simulink model "RM3ControlSim"  (R2015b)
settings: Solver=ode4  StartTime=0  StopTime=400  FixedStep=0.1  MaxStep=0.1  RelTol=1e-3
values from neighbouring files (symbols this model uses):
  simu = simulationClass()    [wecSimInputFile.m]
  waves = waveClass('irregular')    [wecSimInputFile.m]
undefined symbols (not defined in the file or in its folder): body, constraint, plant, pto, X, Y, Z
libraries: nesl_utility x72, vrlib x24, sm_lib x24, WECSim_Lib x3, simulink x2
(part 5 of 6)

== system RM3ControlSim/Rigid Body/Hydrodynamic Body/Morrison Element and ViscousDampingForceCalculation/Morrison Element Variant Subsystem/Morrison Element On/Regular Wave Morison Force/MorrisonElements/OrbitalVelocity ==
  Disp : Inport
  Time : Inport  Port=2
  MATLAB Function : MATLAB Function  TreatAsAtomicUnit=on
  WaveAmp : Constant  Value=waves.A(1,:)
  WaveFreq : Constant  Value=waves.w(1,:)
  WaveNumber : Constant  Value=waves.k(1,:)
  gravity : Constant  Value=simu.g  VectorParams1D=off
  phase : Constant  Value=0
  rampTime : Constant  Value=simu.rampTime  VectorParams1D=off
  waterDepth : Constant  Value=waves.waterDepth  VectorParams1D=off
  waveDirection : Constant  Value=waves.waveDir  VectorParams1D=off
  u-V : Outport
  w-V : Outport  Port=2
  u-A : Outport  Port=3
  w-A : Outport  Port=4
  v-V : Outport  Port=5
  v-A : Outport  Port=6
  wires:
  MATLAB Function/5(ya) -> v-A/1
  MATLAB Function/1(u) -> u-V/1
  MATLAB Function/2(v) -> v-V/1
  MATLAB Function/6(za) -> w-A/1
  MATLAB Function/4(xa) -> u-A/1
  MATLAB Function/3(w) -> w-V/1
  rampTime/1 -> MATLAB Function/7(rampT)
  waveDirection/1 -> MATLAB Function/8(waveDir)
  waterDepth/1 -> MATLAB Function/9(waterDepth)
  gravity/1 -> MATLAB Function/10(g)
  Time/1 -> MATLAB Function/6(time)
  WaveAmp/1 -> MATLAB Function/4(waveAmp)
  WaveFreq/1 -> MATLAB Function/3(waveFreq)
  WaveNumber/1 -> MATLAB Function/2(waveNumber)
  phase/1 -> MATLAB Function/5(randPhase)
  Disp/1 -> MATLAB Function/1(disp)

== system RM3ControlSim/Rigid Body/Hydrodynamic Body/Morrison Element and ViscousDampingForceCalculation/Morrison Element Variant Subsystem/Morrison Element On/Regular Wave Morison Force/MorrisonElements/Rotation1 ==
  rot1 : Inport
  rot2 : Inport  Port=2
  rot3 : Inport  Port=3
  2 : Product
  3 : Product  Inputs=3
  7 : Product
  8 : Product  Inputs=3
  Combine : Concatenate  NumInputs=3  Mode=Multidimensional array  ConcatenateDimension=2
  Trigonometric Function{,1..2,6,9,11} (6 alike) : Trigonometry  Operator=cos
  Trigonometric Function{3..5,7..8,10} (6 alike) : Trigonometry
  rot11 : Product
  rot12 : Sum
  rot13 : Sum  Inputs=+-
  rot[1,1-3] : Outport
  wires:
  rot13/1 -> Combine/3
  8/1 -> rot13/2
  7/1 -> rot13/1
  Trigonometric Function11/1 -> 8/3
  Trigonometric Function10/1 -> 8/2
  Trigonometric Function9/1 -> 8/1
  Trigonometric Function8/1 -> 7/2
  Trigonometric Function7/1 -> 7/1
  rot1/1 -> Trigonometric Function7/1, Trigonometric Function9/1, Trigonometric Function4/1, Trigonometric Function2/1
  rot3/1 -> Trigonometric Function8/1, Trigonometric Function11/1, Trigonometric Function6/1, Trigonometric Function3/1, Trigonometric Function1/1
  rot2/1 -> Trigonometric Function10/1, Trigonometric Function5/1, Trigonometric Function/1
  Combine/1 -> rot[1,1-3]/1
  rot12/1 -> Combine/2
  3/1 -> rot12/2
  2/1 -> rot12/1
  Trigonometric Function6/1 -> 3/3
  Trigonometric Function5/1 -> 3/2
  Trigonometric Function4/1 -> 3/1
  Trigonometric Function3/1 -> 2/2
  Trigonometric Function2/1 -> 2/1
  rot11/1 -> Combine/1
  Trigonometric Function1/1 -> rot11/2
  Trigonometric Function/1 -> rot11/1

== system RM3ControlSim/Rigid Body/Hydrodynamic Body/Morrison Element and ViscousDampingForceCalculation/Morrison Element Variant Subsystem/Morrison Element On/Regular Wave Morison Force/MorrisonElements/Rotation2 ==
  rot1 : Inport
  rot2 : Inport  Port=2
  rot3 : Inport  Port=3
  2 : Product
  3 : Product  Inputs=3
  7 : Product
  8 : Product  Inputs=3
  Combine : Concatenate  NumInputs=3  Mode=Multidimensional array  ConcatenateDimension=2
  Gain : Gain  Gain=-1
  Trigonometric Function{,2..3,8..9} (5 alike) : Trigonometry  Operator=cos
  Trigonometric Function{1,4..7,10..11} (7 alike) : Trigonometry
  rot11 : Product
  rot12 : Sum  Inputs=+-
  rot13 : Sum
  rot[2,1-3] : Outport
  wires:
  Gain/1 -> rot11/1
  rot13/1 -> Combine/3
  8/1 -> rot13/2
  7/1 -> rot13/1
  Trigonometric Function11/1 -> 8/3
  Trigonometric Function10/1 -> 8/2
  Trigonometric Function9/1 -> 8/1
  Trigonometric Function8/1 -> 7/2
  Trigonometric Function7/1 -> 7/1
  rot1/1 -> Trigonometric Function7/1, Trigonometric Function9/1, Trigonometric Function4/1, Trigonometric Function2/1
  rot3/1 -> Trigonometric Function8/1, Trigonometric Function11/1, Trigonometric Function6/1, Trigonometric Function3/1, Trigonometric Function1/1
  rot2/1 -> Trigonometric Function10/1, Trigonometric Function5/1, Trigonometric Function/1
  Combine/1 -> rot[2,1-3]/1
  rot12/1 -> Combine/2
  3/1 -> rot12/2
  2/1 -> rot12/1
  Trigonometric Function6/1 -> 3/3
  Trigonometric Function5/1 -> 3/2
  Trigonometric Function4/1 -> 3/1
  Trigonometric Function3/1 -> 2/2
  Trigonometric Function2/1 -> 2/1
  rot11/1 -> Combine/1
  Trigonometric Function1/1 -> rot11/2
  Trigonometric Function/1 -> Gain/1

== system RM3ControlSim/Rigid Body/Hydrodynamic Body/Morrison Element and ViscousDampingForceCalculation/Morrison Element Variant Subsystem/Morrison Element On/Regular Wave Morison Force/MorrisonElements/Rotation3 ==
  rot1 : Inport
  rot2 : Inport  Port=2
  2 : Product
  7 : Product
  Combine : Concatenate  NumInputs=3  Mode=Multidimensional array  ConcatenateDimension=2
  Gain1 : Gain  Gain=-1
  TrigFun1 : Trigonometry
  TrigFun2 : Trigonometry
  TrigFun3 : Trigonometry  Operator=cos
  TrigFun4 : Trigonometry  Operator=cos
  TrigFun5 : Trigonometry  Operator=cos
  rot[3,1-3] : Outport
  wires:
  Gain1/1 -> 2/1
  TrigFun2/1 -> Gain1/1
  7/1 -> Combine/3
  rot1/1 -> TrigFun4/1, TrigFun2/1
  TrigFun5/1 -> 7/2
  TrigFun4/1 -> 7/1
  rot2/1 -> TrigFun1/1, TrigFun3/1, TrigFun5/1
  Combine/1 -> rot[3,1-3]/1
  2/1 -> Combine/2
  TrigFun3/1 -> 2/2
  TrigFun1/1 -> Combine/1

== system RM3ControlSim/Rigid Body1/Hydrodynamic Body/Morrison Element and ViscousDampingForceCalculation/Morrison Element Variant Subsystem/Morrison Element On/Irregular Wave Morison Force/MorrisonElements/MorisonElementIrregular ==
  Disp : Inport
  waves.kirr : Inport  Port=2  Partition=on  PartitionDimension=1  PartitionWidth=1
  waves.w : Inport  Port=3  Partition=on  PartitionDimension=1  PartitionWidth=1
  waves.A : Inport  Port=4  Partition=on  PartitionDimension=1  PartitionWidth=1
  waves.RandPhase : Inport  Port=5  Partition=on  PartitionDimension=1  PartitionWidth=1
  Time : Inport  Port=6
  For Each : ForEach  DisableCoverage=on  IndexMode=One-based
  MATLAB Function : MATLAB Function  TreatAsAtomicUnit=on
  gravity : Constant  Value=simu.g  VectorParams1D=off
  rampTime : Constant  Value=simu.rampTime  VectorParams1D=off
  waterDepth : Constant  Value=waves.waterDepth  VectorParams1D=off
  waveDirection : Constant  Value=waves.waveDir  VectorParams1D=off
  u-V : Outport  ConcatenationDimension=1
  w-V : Outport  Port=2  ConcatenationDimension=1
  x-A : Outport  Port=3  ConcatenationDimension=1
  w-A : Outport  Port=4  ConcatenationDimension=1
  v-V : Outport  Port=5  ConcatenationDimension=1
  y-A : Outport  Port=6  ConcatenationDimension=1
  wires:
  MATLAB Function/3(w) -> w-V/1
  MATLAB Function/4(xa) -> x-A/1
  MATLAB Function/6(za) -> w-A/1
  MATLAB Function/5(ya) -> y-A/1
  MATLAB Function/2(v) -> v-V/1
  Time/1 -> MATLAB Function/6(time)
  waves.kirr/1 -> MATLAB Function/2(waveNumber)
  MATLAB Function/1(u) -> u-V/1
  waves.RandPhase/1 -> MATLAB Function/5(randPhase)
  waves.A/1 -> MATLAB Function/4(waveAmp)
  waves.w/1 -> MATLAB Function/3(waveFreq)
  Disp/1 -> MATLAB Function/1(disp)
  rampTime/1 -> MATLAB Function/7(rampT)
  waveDirection/1 -> MATLAB Function/8(waveDir)
  waterDepth/1 -> MATLAB Function/9(waterDepth)
  gravity/1 -> MATLAB Function/10(g)

== system RM3ControlSim/Rigid Body1/Hydrodynamic Body/Morrison Element and ViscousDampingForceCalculation/Morrison Element Variant Subsystem/Morrison Element On/Irregular Wave Morison Force/MorrisonElements/Rotation1 ==
  rot1 : Inport
  rot2 : Inport  Port=2
  rot3 : Inport  Port=3
  2 : Product
  3 : Product  Inputs=3
  7 : Product
  8 : Product  Inputs=3
  Combine : Concatenate  NumInputs=3  Mode=Multidimensional array  ConcatenateDimension=2
  Trigonometric Function{,1..2,6,9,11} (6 alike) : Trigonometry  Operator=cos
  Trigonometric Function{3..5,7..8,10} (6 alike) : Trigonometry
  rot11 : Product
  rot12 : Sum
  rot13 : Sum  Inputs=+-
  rot[1,1-3] : Outport
  wires:
  rot13/1 -> Combine/3
  8/1 -> rot13/2
  7/1 -> rot13/1
  Trigonometric Function11/1 -> 8/3
  Trigonometric Function10/1 -> 8/2
  Trigonometric Function9/1 -> 8/1
  Trigonometric Function8/1 -> 7/2
  Trigonometric Function7/1 -> 7/1
  rot1/1 -> Trigonometric Function7/1, Trigonometric Function9/1, Trigonometric Function4/1, Trigonometric Function2/1
  rot3/1 -> Trigonometric Function8/1, Trigonometric Function11/1, Trigonometric Function6/1, Trigonometric Function3/1, Trigonometric Function1/1
  rot2/1 -> Trigonometric Function10/1, Trigonometric Function5/1, Trigonometric Function/1
  Combine/1 -> rot[1,1-3]/1
  rot12/1 -> Combine/2
  3/1 -> rot12/2
  2/1 -> rot12/1
  Trigonometric Function6/1 -> 3/3
  Trigonometric Function5/1 -> 3/2
  Trigonometric Function4/1 -> 3/1
  Trigonometric Function3/1 -> 2/2
  Trigonometric Function2/1 -> 2/1
  rot11/1 -> Combine/1
  Trigonometric Function1/1 -> rot11/2
  Trigonometric Function/1 -> rot11/1

== system RM3ControlSim/Rigid Body1/Hydrodynamic Body/Morrison Element and ViscousDampingForceCalculation/Morrison Element Variant Subsystem/Morrison Element On/Irregular Wave Morison Force/MorrisonElements/Rotation2 ==
  rot1 : Inport
  rot2 : Inport  Port=2
  rot3 : Inport  Port=3
  2 : Product
  3 : Product  Inputs=3
  7 : Product
  8 : Product  Inputs=3
  Combine : Concatenate  NumInputs=3  Mode=Multidimensional array  ConcatenateDimension=2
  Gain : Gain  Gain=-1
  Trigonometric Function{,2..3,8..9} (5 alike) : Trigonometry  Operator=cos
  Trigonometric Function{1,4..7,10..11} (7 alike) : Trigonometry
  rot11 : Product
  rot12 : Sum  Inputs=+-
  rot13 : Sum
  rot[2,1-3] : Outport
  wires:
  Gain/1 -> rot11/1
  rot13/1 -> Combine/3
  8/1 -> rot13/2
  7/1 -> rot13/1
  Trigonometric Function11/1 -> 8/3
  Trigonometric Function10/1 -> 8/2
  Trigonometric Function9/1 -> 8/1
  Trigonometric Function8/1 -> 7/2
  Trigonometric Function7/1 -> 7/1
  rot1/1 -> Trigonometric Function7/1, Trigonometric Function9/1, Trigonometric Function4/1, Trigonometric Function2/1
  rot3/1 -> Trigonometric Function8/1, Trigonometric Function11/1, Trigonometric Function6/1, Trigonometric Function3/1, Trigonometric Function1/1
  rot2/1 -> Trigonometric Function10/1, Trigonometric Function5/1, Trigonometric Function/1
  Combine/1 -> rot[2,1-3]/1
  rot12/1 -> Combine/2
  3/1 -> rot12/2
  2/1 -> rot12/1
  Trigonometric Function6/1 -> 3/3
  Trigonometric Function5/1 -> 3/2
  Trigonometric Function4/1 -> 3/1
  Trigonometric Function3/1 -> 2/2
  Trigonometric Function2/1 -> 2/1
  rot11/1 -> Combine/1
  Trigonometric Function1/1 -> rot11/2
  Trigonometric Function/1 -> Gain/1

== system RM3ControlSim/Rigid Body1/Hydrodynamic Body/Morrison Element and ViscousDampingForceCalculation/Morrison Element Variant Subsystem/Morrison Element On/Irregular Wave Morison Force/MorrisonElements/Rotation3 ==
  rot1 : Inport
  rot2 : Inport  Port=2
  2 : Product
  7 : Product
  Combine : Concatenate  NumInputs=3  Mode=Multidimensional array  ConcatenateDimension=2
  Gain1 : Gain  Gain=-1
  TrigFun1 : Trigonometry
  TrigFun2 : Trigonometry
  TrigFun3 : Trigonometry  Operator=cos
  TrigFun4 : Trigonometry  Operator=cos
  TrigFun5 : Trigonometry  Operator=cos
  rot[3,1-3] : Outport
  wires:
  Gain1/1 -> 2/1
  TrigFun2/1 -> Gain1/1
  7/1 -> Combine/3
  rot1/1 -> TrigFun4/1, TrigFun2/1
  TrigFun5/1 -> 7/2
  TrigFun4/1 -> 7/1
  rot2/1 -> TrigFun1/1, TrigFun3/1, TrigFun5/1
  Combine/1 -> rot[3,1-3]/1
  2/1 -> Combine/2
  TrigFun3/1 -> 2/2
  TrigFun1/1 -> Combine/1

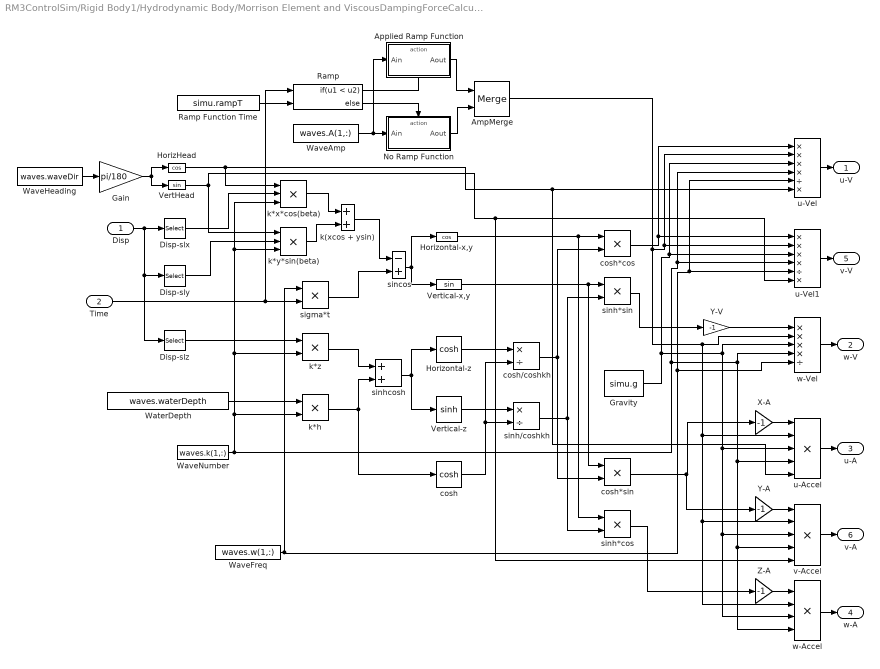
== system RM3ControlSim/Rigid Body1/Hydrodynamic Body/Morrison Element and ViscousDampingForceCalculation/Morrison Element Variant Subsystem/Morrison Element On/No Wave Morison Force/MorrisonElements/OrbitalVelocity ==
  Disp : Inport
  Time : Inport  Port=2
  AmpMerge : Merge
  Applied Ramp Function : Subsystem  TreatAsAtomicUnit=on
  Disp-slx : Selector  InputPortWidth=3  IndexOptions=Index vector (dialog)  Indices=[1]  OutputSizes=1
  Disp-sly : Selector  InputPortWidth=3  IndexOptions=Index vector (dialog)  Indices=[2]  OutputSizes=1
  Disp-slz : Selector  InputPortWidth=3  IndexOptions=Index vector (dialog)  Indices=[3]  OutputSizes=1
  Gain : Gain  Gain=pi/180
  Gravity : Constant  Value=simu.g
  HorizHead : Trigonometry  Operator=cos
  Horizontal-x,y : Trigonometry  Operator=cos
  Horizontal-z : Trigonometry  Operator=cosh
  No Ramp Function : Subsystem  TreatAsAtomicUnit=on
  Ramp : If  NumInputs=2  IfExpression=u1 < u2
  Ramp Function Time : Constant  Value=simu.rampT
  VertHead : Trigonometry
  Vertical-x,y : Trigonometry
  Vertical-z : Trigonometry  Operator=sinh
  WaterDepth : Constant  Value=waves.waterDepth
  WaveAmp : Constant  Value=waves.A(1,:)
  WaveFreq : Constant  Value=waves.w(1,:)
  WaveHeading : Constant  Value=waves.waveDir
  WaveNumber : Constant  Value=waves.k(1,:)
  X-A : Gain  Gain=-1
  Y-A : Gain  Gain=-1
  Y-V : Gain  Gain=-1
  Z-A : Gain  Gain=-1
  cosh : Trigonometry  Operator=cosh
  cosh*cos : Product  Inputs=**
  cosh*sin : Product  Inputs=**
  cosh/coshkh : Product  Inputs=*/
  k(xcos + ysin) : Sum
  k*h : Product
  k*x*cos(beta) : Product  Inputs=3
  k*y*sin(beta) : Product  Inputs=3
  k*z : Product
  sigma*t : Product
  sincos : Sum  Inputs=-+
  sinh*cos : Product  Inputs=**
  sinh*sin : Product  Inputs=**
  sinh/coshkh : Product  Inputs=*/
  sinhcosh : Sum
  u-Accel : Product  Inputs=*****
  u-Vel : Product  Inputs=****/*
  u-Vel1 : Product  Inputs=****/*
  v-Accel : Product  Inputs=*****
  w-Accel : Product  Inputs=****
  w-Vel : Product  Inputs=****/
  u-V : Outport
  w-V : Outport  Port=2
  u-A : Outport  Port=3
  w-A : Outport  Port=4
  v-V : Outport  Port=5
  v-A : Outport  Port=6
  wires:
  v-Accel/1 -> v-A/1
  Y-A/1 -> v-Accel/1
  u-Vel/1 -> u-V/1
  u-Vel1/1 -> v-V/1
  k(xcos + ysin)/1 -> sincos/1
  k*x*cos(beta)/1 -> k(xcos + ysin)/1
  k*y*sin(beta)/1 -> k(xcos + ysin)/2
  VertHead/1 -> v-Accel/5, u-Vel1/6, k*y*sin(beta)/1
  HorizHead/1 -> k*x*cos(beta)/1, u-Vel/6, u-Accel/5
  Disp-slx/1 -> k*x*cos(beta)/2
  Gain/1 -> VertHead/1, HorizHead/1
  WaveHeading/1 -> Gain/1
  WaveAmp/1 -> No Ramp Function/1(Ain), Applied Ramp Function/1(Ain)
  WaveFreq/1 -> sigma*t/1, u-Vel/5, u-Vel1/5, w-Vel/5
  Disp-slz/1 -> k*z/1
  Applied Ramp Function/1(Aout) -> AmpMerge/1
  No Ramp Function/1(Aout) -> AmpMerge/2
  Time/1 -> sigma*t/2, Ramp/1
  Ramp/1 -> Applied Ramp Function/Action
  Ramp/2 -> No Ramp Function/Action
  Ramp Function Time/1 -> Ramp/2
  sinh*cos/1 -> Z-A/1
  cosh*sin/1 -> X-A/1, Y-A/1
  w-Accel/1 -> w-A/1
  u-Accel/1 -> u-A/1
  w-Vel/1 -> w-V/1
  Z-A/1 -> w-Accel/1
  X-A/1 -> u-Accel/1
  Y-V/1 -> w-Vel/1
  sinh*sin/1 -> Y-V/1
  Gravity/1 -> u-Vel/3, u-Vel1/3, u-Accel/3, w-Accel/3, v-Accel/3, w-Vel/3
  AmpMerge/1 -> u-Vel/2, u-Vel1/2, u-Accel/2, v-Accel/2, w-Accel/2, w-Vel/2
  cosh*cos/1 -> u-Vel/1, u-Vel1/1
  Disp-sly/1 -> k*y*sin(beta)/2
  cosh/coshkh/1 -> cosh*sin/2, cosh*cos/2
  Horizontal-x,y/1 -> cosh*cos/1, sinh*cos/1
  sinh/coshkh/1 -> sinh*sin/2, sinh*cos/2
  Vertical-x,y/1 -> sinh*sin/1, cosh*sin/1
  Vertical-z/1 -> sinh/coshkh/1
  cosh/1 -> cosh/coshkh/2, sinh/coshkh/2
  Horizontal-z/1 -> cosh/coshkh/1
  sinhcosh/1 -> Horizontal-z/1, Vertical-z/1
  k*h/1 -> sinhcosh/2, cosh/1
  k*z/1 -> sinhcosh/1
  sincos/1 -> Horizontal-x,y/1, Vertical-x,y/1
  sigma*t/1 -> sincos/2
  WaterDepth/1 -> k*h/1
  WaveNumber/1 -> u-Vel/4, u-Vel1/4, u-Accel/4, w-Accel/4, v-Accel/4, w-Vel/4, k*x*cos(beta)/3, k*y*sin(beta)/3, k*z/2, k*h/2
  Disp/1 -> Disp-slx/1, Disp-sly/1, Disp-slz/1

== system RM3ControlSim/Rigid Body1/Hydrodynamic Body/Morrison Element and ViscousDampingForceCalculation/Morrison Element Variant Subsystem/Morrison Element On/No Wave Morison Force/MorrisonElements/Rotation1 ==
  rot1 : Inport
  rot2 : Inport  Port=2
  rot3 : Inport  Port=3
  2 : Product
  3 : Product  Inputs=3
  7 : Product
  8 : Product  Inputs=3
  Combine : Concatenate  NumInputs=3  Mode=Multidimensional array  ConcatenateDimension=2
  Trigonometric Function{,1..2,6,9,11} (6 alike) : Trigonometry  Operator=cos
  Trigonometric Function{3..5,7..8,10} (6 alike) : Trigonometry
  rot11 : Product
  rot12 : Sum
  rot13 : Sum  Inputs=+-
  rot[1,1-3] : Outport
  wires:
  rot13/1 -> Combine/3
  8/1 -> rot13/2
  7/1 -> rot13/1
  Trigonometric Function11/1 -> 8/3
  Trigonometric Function10/1 -> 8/2
  Trigonometric Function9/1 -> 8/1
  Trigonometric Function8/1 -> 7/2
  Trigonometric Function7/1 -> 7/1
  rot1/1 -> Trigonometric Function7/1, Trigonometric Function9/1, Trigonometric Function4/1, Trigonometric Function2/1
  rot3/1 -> Trigonometric Function8/1, Trigonometric Function11/1, Trigonometric Function6/1, Trigonometric Function3/1, Trigonometric Function1/1
  rot2/1 -> Trigonometric Function10/1, Trigonometric Function5/1, Trigonometric Function/1
  Combine/1 -> rot[1,1-3]/1
  rot12/1 -> Combine/2
  3/1 -> rot12/2
  2/1 -> rot12/1
  Trigonometric Function6/1 -> 3/3
  Trigonometric Function5/1 -> 3/2
  Trigonometric Function4/1 -> 3/1
  Trigonometric Function3/1 -> 2/2
  Trigonometric Function2/1 -> 2/1
  rot11/1 -> Combine/1
  Trigonometric Function1/1 -> rot11/2
  Trigonometric Function/1 -> rot11/1

== system RM3ControlSim/Rigid Body1/Hydrodynamic Body/Morrison Element and ViscousDampingForceCalculation/Morrison Element Variant Subsystem/Morrison Element On/No Wave Morison Force/MorrisonElements/Rotation2 ==
  rot1 : Inport
  rot2 : Inport  Port=2
  rot3 : Inport  Port=3
  2 : Product
  3 : Product  Inputs=3
  7 : Product
  8 : Product  Inputs=3
  Combine : Concatenate  NumInputs=3  Mode=Multidimensional array  ConcatenateDimension=2
  Gain : Gain  Gain=-1
  Trigonometric Function{,2..3,8..9} (5 alike) : Trigonometry  Operator=cos
  Trigonometric Function{1,4..7,10..11} (7 alike) : Trigonometry
  rot11 : Product
  rot12 : Sum  Inputs=+-
  rot13 : Sum
  rot[2,1-3] : Outport
  wires:
  Gain/1 -> rot11/1
  rot13/1 -> Combine/3
  8/1 -> rot13/2
  7/1 -> rot13/1
  Trigonometric Function11/1 -> 8/3
  Trigonometric Function10/1 -> 8/2
  Trigonometric Function9/1 -> 8/1
  Trigonometric Function8/1 -> 7/2
  Trigonometric Function7/1 -> 7/1
  rot1/1 -> Trigonometric Function7/1, Trigonometric Function9/1, Trigonometric Function4/1, Trigonometric Function2/1
  rot3/1 -> Trigonometric Function8/1, Trigonometric Function11/1, Trigonometric Function6/1, Trigonometric Function3/1, Trigonometric Function1/1
  rot2/1 -> Trigonometric Function10/1, Trigonometric Function5/1, Trigonometric Function/1
  Combine/1 -> rot[2,1-3]/1
  rot12/1 -> Combine/2
  3/1 -> rot12/2
  2/1 -> rot12/1
  Trigonometric Function6/1 -> 3/3
  Trigonometric Function5/1 -> 3/2
  Trigonometric Function4/1 -> 3/1
  Trigonometric Function3/1 -> 2/2
  Trigonometric Function2/1 -> 2/1
  rot11/1 -> Combine/1
  Trigonometric Function1/1 -> rot11/2
  Trigonometric Function/1 -> Gain/1

== system RM3ControlSim/Rigid Body1/Hydrodynamic Body/Morrison Element and ViscousDampingForceCalculation/Morrison Element Variant Subsystem/Morrison Element On/No Wave Morison Force/MorrisonElements/Rotation3 ==
  rot1 : Inport
  rot2 : Inport  Port=2
  2 : Product
  7 : Product
  Combine : Concatenate  NumInputs=3  Mode=Multidimensional array  ConcatenateDimension=2
  Gain1 : Gain  Gain=-1
  TrigFun1 : Trigonometry
  TrigFun2 : Trigonometry
  TrigFun3 : Trigonometry  Operator=cos
  TrigFun4 : Trigonometry  Operator=cos
  TrigFun5 : Trigonometry  Operator=cos
  rot[3,1-3] : Outport
  wires:
  Gain1/1 -> 2/1
  TrigFun2/1 -> Gain1/1
  7/1 -> Combine/3
  rot1/1 -> TrigFun4/1, TrigFun2/1
  TrigFun5/1 -> 7/2
  TrigFun4/1 -> 7/1
  rot2/1 -> TrigFun1/1, TrigFun3/1, TrigFun5/1
  Combine/1 -> rot[3,1-3]/1
  2/1 -> Combine/2
  TrigFun3/1 -> 2/2
  TrigFun1/1 -> Combine/1

== system RM3ControlSim/Rigid Body1/Hydrodynamic Body/Morrison Element and ViscousDampingForceCalculation/Morrison Element Variant Subsystem/Morrison Element On/Regular Wave Morison Force/MorrisonElements/OrbitalVelocity ==
  Disp : Inport
  Time : Inport  Port=2
  MATLAB Function : MATLAB Function  TreatAsAtomicUnit=on
  WaveAmp : Constant  Value=waves.A(1,:)
  WaveFreq : Constant  Value=waves.w(1,:)
  WaveNumber : Constant  Value=waves.k(1,:)
  gravity : Constant  Value=simu.g  VectorParams1D=off
  phase : Constant  Value=0
  rampTime : Constant  Value=simu.rampTime  VectorParams1D=off
  waterDepth : Constant  Value=waves.waterDepth  VectorParams1D=off
  waveDirection : Constant  Value=waves.waveDir  VectorParams1D=off
  u-V : Outport
  w-V : Outport  Port=2
  u-A : Outport  Port=3
  w-A : Outport  Port=4
  v-V : Outport  Port=5
  v-A : Outport  Port=6
  wires:
  MATLAB Function/5(ya) -> v-A/1
  MATLAB Function/1(u) -> u-V/1
  MATLAB Function/2(v) -> v-V/1
  MATLAB Function/6(za) -> w-A/1
  MATLAB Function/4(xa) -> u-A/1
  MATLAB Function/3(w) -> w-V/1
  rampTime/1 -> MATLAB Function/7(rampT)
  waveDirection/1 -> MATLAB Function/8(waveDir)
  waterDepth/1 -> MATLAB Function/9(waterDepth)
  gravity/1 -> MATLAB Function/10(g)
  Time/1 -> MATLAB Function/6(time)
  WaveAmp/1 -> MATLAB Function/4(waveAmp)
  WaveFreq/1 -> MATLAB Function/3(waveFreq)
  WaveNumber/1 -> MATLAB Function/2(waveNumber)
  phase/1 -> MATLAB Function/5(randPhase)
  Disp/1 -> MATLAB Function/1(disp)

== system RM3ControlSim/Rigid Body1/Hydrodynamic Body/Morrison Element and ViscousDampingForceCalculation/Morrison Element Variant Subsystem/Morrison Element On/Regular Wave Morison Force/MorrisonElements/Rotation1 ==
  rot1 : Inport
  rot2 : Inport  Port=2
  rot3 : Inport  Port=3
  2 : Product
  3 : Product  Inputs=3
  7 : Product
  8 : Product  Inputs=3
  Combine : Concatenate  NumInputs=3  Mode=Multidimensional array  ConcatenateDimension=2
  Trigonometric Function{,1..2,6,9,11} (6 alike) : Trigonometry  Operator=cos
  Trigonometric Function{3..5,7..8,10} (6 alike) : Trigonometry
  rot11 : Product
  rot12 : Sum
  rot13 : Sum  Inputs=+-
  rot[1,1-3] : Outport
  wires:
  rot13/1 -> Combine/3
  8/1 -> rot13/2
  7/1 -> rot13/1
  Trigonometric Function11/1 -> 8/3
  Trigonometric Function10/1 -> 8/2
  Trigonometric Function9/1 -> 8/1
  Trigonometric Function8/1 -> 7/2
  Trigonometric Function7/1 -> 7/1
  rot1/1 -> Trigonometric Function7/1, Trigonometric Function9/1, Trigonometric Function4/1, Trigonometric Function2/1
  rot3/1 -> Trigonometric Function8/1, Trigonometric Function11/1, Trigonometric Function6/1, Trigonometric Function3/1, Trigonometric Function1/1
  rot2/1 -> Trigonometric Function10/1, Trigonometric Function5/1, Trigonometric Function/1
  Combine/1 -> rot[1,1-3]/1
  rot12/1 -> Combine/2
  3/1 -> rot12/2
  2/1 -> rot12/1
  Trigonometric Function6/1 -> 3/3
  Trigonometric Function5/1 -> 3/2
  Trigonometric Function4/1 -> 3/1
  Trigonometric Function3/1 -> 2/2
  Trigonometric Function2/1 -> 2/1
  rot11/1 -> Combine/1
  Trigonometric Function1/1 -> rot11/2
  Trigonometric Function/1 -> rot11/1

== system RM3ControlSim/Rigid Body1/Hydrodynamic Body/Morrison Element and ViscousDampingForceCalculation/Morrison Element Variant Subsystem/Morrison Element On/Regular Wave Morison Force/MorrisonElements/Rotation2 ==
  rot1 : Inport
  rot2 : Inport  Port=2
  rot3 : Inport  Port=3
  2 : Product
  3 : Product  Inputs=3
  7 : Product
  8 : Product  Inputs=3
  Combine : Concatenate  NumInputs=3  Mode=Multidimensional array  ConcatenateDimension=2
  Gain : Gain  Gain=-1
  Trigonometric Function{,2..3,8..9} (5 alike) : Trigonometry  Operator=cos
  Trigonometric Function{1,4..7,10..11} (7 alike) : Trigonometry
  rot11 : Product
  rot12 : Sum  Inputs=+-
  rot13 : Sum
  rot[2,1-3] : Outport
  wires:
  Gain/1 -> rot11/1
  rot13/1 -> Combine/3
  8/1 -> rot13/2
  7/1 -> rot13/1
  Trigonometric Function11/1 -> 8/3
  Trigonometric Function10/1 -> 8/2
  Trigonometric Function9/1 -> 8/1
  Trigonometric Function8/1 -> 7/2
  Trigonometric Function7/1 -> 7/1
  rot1/1 -> Trigonometric Function7/1, Trigonometric Function9/1, Trigonometric Function4/1, Trigonometric Function2/1
  rot3/1 -> Trigonometric Function8/1, Trigonometric Function11/1, Trigonometric Function6/1, Trigonometric Function3/1, Trigonometric Function1/1
  rot2/1 -> Trigonometric Function10/1, Trigonometric Function5/1, Trigonometric Function/1
  Combine/1 -> rot[2,1-3]/1
  rot12/1 -> Combine/2
  3/1 -> rot12/2
  2/1 -> rot12/1
  Trigonometric Function6/1 -> 3/3
  Trigonometric Function5/1 -> 3/2
  Trigonometric Function4/1 -> 3/1
  Trigonometric Function3/1 -> 2/2
  Trigonometric Function2/1 -> 2/1
  rot11/1 -> Combine/1
  Trigonometric Function1/1 -> rot11/2
  Trigonometric Function/1 -> Gain/1

== system RM3ControlSim/Rigid Body1/Hydrodynamic Body/Morrison Element and ViscousDampingForceCalculation/Morrison Element Variant Subsystem/Morrison Element On/Regular Wave Morison Force/MorrisonElements/Rotation3 ==
  rot1 : Inport
  rot2 : Inport  Port=2
  2 : Product
  7 : Product
  Combine : Concatenate  NumInputs=3  Mode=Multidimensional array  ConcatenateDimension=2
  Gain1 : Gain  Gain=-1
  TrigFun1 : Trigonometry
  TrigFun2 : Trigonometry
  TrigFun3 : Trigonometry  Operator=cos
  TrigFun4 : Trigonometry  Operator=cos
  TrigFun5 : Trigonometry  Operator=cos
  rot[3,1-3] : Outport
  wires:
  Gain1/1 -> 2/1
  TrigFun2/1 -> Gain1/1
  7/1 -> Combine/3
  rot1/1 -> TrigFun4/1, TrigFun2/1
  TrigFun5/1 -> 7/2
  TrigFun4/1 -> 7/1
  rot2/1 -> TrigFun1/1, TrigFun3/1, TrigFun5/1
  Combine/1 -> rot[3,1-3]/1
  2/1 -> Combine/2
  TrigFun3/1 -> 2/2
  TrigFun1/1 -> Combine/1

== system RM3ControlSim/Rigid Body/Hydrodynamic Body/Morrison Element and ViscousDampingForceCalculation/Morrison Element Variant Subsystem/Morrison Element On/No Wave Morison Force/MorrisonElements/OrbitalVelocity/Applied Ramp Function ==
  Ain : Inport
  Action Port : ActionPort
  Add : Sum
  Constant : Constant  Value=2
  Constant1 : Constant
  Divide : Product  Inputs=**/
  Sine Wave : Sin  Frequency=pi/simu.rampT  Phase=pi+pi/2  SampleTime=0
  Aout : Outport
  wires:
  Add/1 -> Divide/2
  Sine Wave/1 -> Add/2
  Constant1/1 -> Add/1
  Constant/1 -> Divide/3
  Divide/1 -> Aout/1
  Ain/1 -> Divide/1

== system RM3ControlSim/Rigid Body/Hydrodynamic Body/Morrison Element and ViscousDampingForceCalculation/Morrison Element Variant Subsystem/Morrison Element On/No Wave Morison Force/MorrisonElements/OrbitalVelocity/No Ramp Function ==
  Ain : Inport
  Action Port : ActionPort
  Aout : Outport
  wires:
  Ain/1 -> Aout/1

== system RM3ControlSim/Rigid Body1/Hydrodynamic Body/Morrison Element and ViscousDampingForceCalculation/Morrison Element Variant Subsystem/Morrison Element On/No Wave Morison Force/MorrisonElements/OrbitalVelocity/Applied Ramp Function ==
  Ain : Inport
  Action Port : ActionPort
  Add : Sum
  Constant : Constant  Value=2
  Constant1 : Constant
  Divide : Product  Inputs=**/
  Sine Wave : Sin  Frequency=pi/simu.rampT  Phase=pi+pi/2  SampleTime=0
  Aout : Outport
  wires:
  Add/1 -> Divide/2
  Sine Wave/1 -> Add/2
  Constant1/1 -> Add/1
  Constant/1 -> Divide/3
  Divide/1 -> Aout/1
  Ain/1 -> Divide/1

== system RM3ControlSim/Rigid Body1/Hydrodynamic Body/Morrison Element and ViscousDampingForceCalculation/Morrison Element Variant Subsystem/Morrison Element On/No Wave Morison Force/MorrisonElements/OrbitalVelocity/No Ramp Function ==
  Ain : Inport
  Action Port : ActionPort
  Aout : Outport
  wires:
  Ain/1 -> Aout/1

== matlab function RM3ControlSim/Rigid Body/Hydrodynamic Body/Hydrostatic Restoring Force Calculation/Linear and Nonlinear Restoring Force Variant Subsystem/Nonlinear Hydrostatic Restoring Force/Diffarction and Excitation Forces1 ==
  data: x input; elv input; center input; f output; tnorm input; area input; rho input; g input; cg input; p output; dt input; dtFe input; t input
function [f,p]  = nonLinearBuoyancy(x,elv,center,tnorm,area,rho,g,cg,dt,dtFe,t)
% Function to calculate buoyancy force and moment on a triangulated surface
% NOTE: This function assumes that the STL file is imported with its CG at 0,0,0
persistent oldF 
persistent oldP

if isempty(oldF)
    [f,p] = calc_buoyancy(x,elv,center,tnorm,area,rho,g,cg);
    oldF  = f;
    oldP  = p;
else
    if mod(t, dtFe) < dt/2
        [f,p] = calc_buoyancy(x,elv,center,tnorm,area,rho,g,cg);
        oldF  = f;
        oldP  = p;
    else
        f  = oldF;
        p  = oldP;
    end
end
end


function [f,p] = calc_buoyancy(x,elv,center,tnorm,area,rho,g,cg)
% Function to apply translation and rotation and calculate forces

% Compute new tri coords after cog rotation and translation
center = rotateXYZ(center,[1 0 0],x(4));
center = rotateXYZ(center,[0 1 0],x(5));
center = rotateXYZ(center,[0 0 1],x(6));
center = offsetXYZ(center,x);
center = offsetXYZ(center,cg);
% Compute new normal vectors coords after cog rotation
tnorm = rotateXYZ(tnorm,[1 0 0],x(4));
tnorm = rotateXYZ(tnorm,[0 1 0],x(5));
tnorm = rotateXYZ(tnorm,[0 0 1],x(6));

% Calculate the hydrostatic forces
av = tnorm .* [area area area];
[f,p]=fHydrostatic(center,elv,x(1:3)+cg,av,rho,g); 
end

function verts = offsetXYZ(verts,x)
% Function to move the position vertices
verts(:,1) = verts(:,1) + x(1);
verts(:,2) = verts(:,2) + x(2);
verts(:,3) = verts(:,3) + x(3);
end

function xn = rotateXYZ(x,ax,t)
	% Function to rotate a point about an arbitrary axis
	% x: 3-componenet coordiantes
	% ax: axis about which to rotate (must be a vector length 1)
	% t: rotation angle
	% xn: new coordinates after rotation
	rotMat = zeros(3);
	rotMat(1,1) = ax(1)*ax(1)*(1-cos(t))    + cos(t);
	rotMat(1,2) = ax(2)*ax(1)*(1-cos(t))    + ax(3)*sin(t);
	rotMat(1,3) = ax(3)*ax(1)*(1-cos(t))    - ax(2)*sin(t);
	rotMat(2,1) = ax(1)*ax(2)*(1-cos(t))    - ax(3)*sin(t);
	rotMat(2,2) = ax(2)*ax(2)*(1-cos(t))    + cos(t);
	rotMat(2,3) = ax(3)*ax(2)*(1-cos(t))    + ax(1)*sin(t);
	rotMat(3,1) = ax(1)*ax(3)*(1-cos(t))    + ax(2)*sin(t);
	rotMat(3,2) = ax(2)*ax(3)*(1-cos(t))    - ax(1)*sin(t);
	rotMat(3,3) = ax(3)*ax(3)*(1-cos(t))    + cos(t);
	xn = x*rotMat;
end

function [f,p] = fHydrostatic(center,elv,instcg,av,rho,g)
% Function to calculate the force and moment about the cog due to hydrostatic pressure
f = zeros(6,1);

% Zeor out regions above the mean free surface
z=center(:,3); z((z-elv)>0)=0;

% Calculate the hydrostatic pressure at each triangle center
pressureVect = rho*g.*[-z -z -z].*-av;
p = rho*g.*-z;
% Compute force about cog
f(1:3) = sum(pressureVect);

tmp1 = ones(length(center(:,1)),1);
tmp2 = tmp1*instcg';
center2cgVec = center-tmp2;

f(4:6)= sum(cross(center2cgVec,pressureVect));
end

== matlab function RM3ControlSim/Rigid Body/Hydrodynamic Body/Morrison Element and ViscousDampingForceCalculation/Morrison Element Variant Subsystem/Morrison Element On/Irregular Wave Morison Force/MorrisonElements/MorisonElementIrregular/MATLAB Function ==
  data: u output; v output; disp input size=[1 3]; waveNumber input; waveFreq input; waveAmp input; randPhase input; time input; rampT input size=[1 1]; waveDir input size=[1 1]; waterDepth input size=[1 1]; g input size=[1 1]; w output; xa output; ya output; za output
function [u,v,w,xa,ya,za] = calc_orbital_vel(disp, waveNumber, waveFreq, waveAmp, randPhase, time, rampT, waveDir, waterDepth, g)
%#codegen

[u,v,w,xa,ya,za] = orbital_velocity(disp, waveNumber, waveFreq, waveAmp, randPhase, time, rampT, waveDir, waterDepth, g);

== matlab function RM3ControlSim/Rigid Body/Hydrodynamic Body/Morrison Element and ViscousDampingForceCalculation/Morrison Element Variant Subsystem/Morrison Element On/Regular Wave Morison Force/MorrisonElements/OrbitalVelocity/MATLAB Function ==
  data: u output; v output; disp input size=[1 3]; waveNumber input size=[1 1]; waveFreq input size=[1 1]; waveAmp input size=[1 1]; randPhase input; time input; rampT input size=[1 1]; waveDir input size=[1 1]; waterDepth input size=[1 1]; g input size=[1 1]; w output; xa output; ya output; za output
function [u,v,w,xa,ya,za] = calc_orbital_vel(disp, waveNumber, waveFreq, waveAmp, randPhase, time, rampT, waveDir, waterDepth, g)
%#codegen

[u,v,w,xa,ya,za] = orbital_velocity(disp, waveNumber, waveFreq, waveAmp, randPhase, time, rampT, waveDir, waterDepth, g);

== matlab function RM3ControlSim/Rigid Body/Hydrodynamic Body/Nonlinear Wave Elevation/Linear or Instantaneous Free Surface/Instantaneous Water Free Surface  /Instantaneous FS ==
  data: x input; center input; f output; cg input; AH input; w input; dw input; k input; typeNum input; t input; rampT input; phaseRand input; waveDir input; dt input; dtFe input
function f  = waveElevation(x,center,cg,AH,w,dw,k,typeNum,t,rampT,phaseRand,waveDir, dt, dtFe)
    % Function to calculate the wave elevation at the ceontroids of triangulated surface
    % NOTE: This function assumes that the STL file is imported with its CG at 0,0,0
    persistent oldElev
    if isempty(oldElev)
        f = calc_elev(x,center,cg,AH,w,dw,k,typeNum,t,rampT,phaseRand, waveDir);
        oldElev = f;
    else
        if mod(t, dtFe) < dt/2
            f = calc_elev(x,center,cg,AH,w,dw,k,typeNum,t,rampT,phaseRand, waveDir);
            oldElev = f;
        else
            f = oldElev;
        end
    end
end

function f = calc_elev(x,center,cg,AH,w,dw,k,typeNum,t,rampT,phaseRand,waveDir)
    % Function to rotate and translate body and call wave elevation function at new locations 
    
    % Compute new tri center coords after cog rotation and translation
    center = rotateXYZ(center,[1 0 0],x(4));
    center = rotateXYZ(center,[0 1 0],x(5));
    center = rotateXYZ(center,[0 0 1],x(6));
    center = offsetXYZ(center,x);
    center = offsetXYZ(center,cg);
    % Calculate the free surface
    f=waveElev(center,AH,w,dw,t,k,rampT,phaseRand,typeNum,waveDir);
end

function verts = offsetXYZ(verts,x)
    % Function to move the position vertices
    verts(:,1) = verts(:,1) + x(1);
    verts(:,2) = verts(:,2) + x(2);
    verts(:,3) = verts(:,3) + x(3);
end

function xn = rotateXYZ(x,ax,t)
	% Function to rotate a point about an arbitrary axis
	% x: 3-component coordinates
	% ax: axis about which to rotate (must be a vector length 1)
	% t: rotation angle
	% xn: new coordinates after rotation
	rotMat = zeros(3);
	rotMat(1,1) = ax(1)*ax(1)*(1-cos(t))    + cos(t);
	rotMat(1,2) = ax(2)*ax(1)*(1-cos(t))    + ax(3)*sin(t);
	rotMat(1,3) = ax(3)*ax(1)*(1-cos(t))    - ax(2)*sin(t);
	rotMat(2,1) = ax(1)*ax(2)*(1-cos(t))    - ax(3)*sin(t);
	rotMat(2,2) = ax(2)*ax(2)*(1-cos(t))    + cos(t);
	rotMat(2,3) = ax(3)*ax(2)*(1-cos(t))    + ax(1)*sin(t);
	rotMat(3,1) = ax(1)*ax(3)*(1-cos(t))    + ax(2)*sin(t);
	rotMat(3,2) = ax(2)*ax(3)*(1-cos(t))    - ax(1)*sin(t);
	rotMat(3,3) = ax(3)*ax(3)*(1-cos(t))    + cos(t);
	xn = x*rotMat;
end

function f=waveElev(center,AH,w,dw,t,k,rampT,phaseRand,typeNum,waveDir)
    % Function to calculate the wave elevation at an array of points
    f = zeros(length(center(:,3)),1);
    cx = center(:,1);
    cy = center(:,2);
    X = cx*cos(waveDir*pi/180) + cy*sin(waveDir*pi/180);
    if typeNum <10
    elseif typeNum <20
        f = AH(1).*cos(k(1).*X-w(1)*t);
    elseif typeNum <30
        tmp=sqrt(AH.*dw);
        tmp1 = ones(1,length(center(:,1)));
        tmp2 = (w.*t+phaseRand)*tmp1;
        tmp3 = cos(k*X'- tmp2);
        f(:,1) = tmp3'*tmp;
    end
    if t<=rampT
        rampF = (1+cos(pi+pi*t/rampT))/2;
        f = f.*rampF;
    end
end

== matlab function RM3ControlSim/Rigid Body1/Hydrodynamic Body/Hydrostatic Restoring Force Calculation/Linear and Nonlinear Restoring Force Variant Subsystem/Nonlinear Hydrostatic Restoring Force/Diffarction and Excitation Forces1 ==
  data: x input; elv input; center input; f output; tnorm input; area input; rho input; g input; cg input; p output; dt input; dtFe input; t input
function [f,p]  = nonLinearBuoyancy(x,elv,center,tnorm,area,rho,g,cg,dt,dtFe,t)
% Function to calculate buoyancy force and moment on a triangulated surface
% NOTE: This function assumes that the STL file is imported with its CG at 0,0,0
persistent oldF 
persistent oldP

if isempty(oldF)
    [f,p] = calc_buoyancy(x,elv,center,tnorm,area,rho,g,cg);
    oldF  = f;
    oldP  = p;
else
    if mod(t, dtFe) < dt/2
        [f,p] = calc_buoyancy(x,elv,center,tnorm,area,rho,g,cg);
        oldF  = f;
        oldP  = p;
    else
        f  = oldF;
        p  = oldP;
    end
end
end


function [f,p] = calc_buoyancy(x,elv,center,tnorm,area,rho,g,cg)
% Function to apply translation and rotation and calculate forces

% Compute new tri coords after cog rotation and translation
center = rotateXYZ(center,[1 0 0],x(4));
center = rotateXYZ(center,[0 1 0],x(5));
center = rotateXYZ(center,[0 0 1],x(6));
center = offsetXYZ(center,x);
center = offsetXYZ(center,cg);
% Compute new normal vectors coords after cog rotation
tnorm = rotateXYZ(tnorm,[1 0 0],x(4));
tnorm = rotateXYZ(tnorm,[0 1 0],x(5));
tnorm = rotateXYZ(tnorm,[0 0 1],x(6));

% Calculate the hydrostatic forces
av = tnorm .* [area area area];
[f,p]=fHydrostatic(center,elv,x(1:3)+cg,av,rho,g); 
end

function verts = offsetXYZ(verts,x)
% Function to move the position vertices
verts(:,1) = verts(:,1) + x(1);
verts(:,2) = verts(:,2) + x(2);
verts(:,3) = verts(:,3) + x(3);
end

function xn = rotateXYZ(x,ax,t)
	% Function to rotate a point about an arbitrary axis
	% x: 3-componenet coordiantes
	% ax: axis about which to rotate (must be a vector length 1)
	% t: rotation angle
	% xn: new coordinates after rotation
	rotMat = zeros(3);
	rotMat(1,1) = ax(1)*ax(1)*(1-cos(t))    + cos(t);
	rotMat(1,2) = ax(2)*ax(1)*(1-cos(t))    + ax(3)*sin(t);
	rotMat(1,3) = ax(3)*ax(1)*(1-cos(t))    - ax(2)*sin(t);
	rotMat(2,1) = ax(1)*ax(2)*(1-cos(t))    - ax(3)*sin(t);
	rotMat(2,2) = ax(2)*ax(2)*(1-cos(t))    + cos(t);
	rotMat(2,3) = ax(3)*ax(2)*(1-cos(t))    + ax(1)*sin(t);
	rotMat(3,1) = ax(1)*ax(3)*(1-cos(t))    + ax(2)*sin(t);
	rotMat(3,2) = ax(2)*ax(3)*(1-cos(t))    - ax(1)*sin(t);
	rotMat(3,3) = ax(3)*ax(3)*(1-cos(t))    + cos(t);
	xn = x*rotMat;
end

function [f,p] = fHydrostatic(center,elv,instcg,av,rho,g)
% Function to calculate the force and moment about the cog due to hydrostatic pressure
f = zeros(6,1);

% Zeor out regions above the mean free surface
z=center(:,3); z((z-elv)>0)=0;

% Calculate the hydrostatic pressure at each triangle center
pressureVect = rho*g.*[-z -z -z].*-av;
p = rho*g.*-z;
% Compute force about cog
f(1:3) = sum(pressureVect);

tmp1 = ones(length(center(:,1)),1);
tmp2 = tmp1*instcg';
center2cgVec = center-tmp2;

f(4:6)= sum(cross(center2cgVec,pressureVect));
end

== matlab function RM3ControlSim/Rigid Body1/Hydrodynamic Body/Morrison Element and ViscousDampingForceCalculation/Morrison Element Variant Subsystem/Morrison Element On/Irregular Wave Morison Force/MorrisonElements/MorisonElementIrregular/MATLAB Function ==
  data: u output; v output; disp input size=[1 3]; waveNumber input; waveFreq input; waveAmp input; randPhase input; time input; rampT input size=[1 1]; waveDir input size=[1 1]; waterDepth input size=[1 1]; g input size=[1 1]; w output; xa output; ya output; za output
function [u,v,w,xa,ya,za] = calc_orbital_vel(disp, waveNumber, waveFreq, waveAmp, randPhase, time, rampT, waveDir, waterDepth, g)
%#codegen

[u,v,w,xa,ya,za] = orbital_velocity(disp, waveNumber, waveFreq, waveAmp, randPhase, time, rampT, waveDir, waterDepth, g);

== matlab function RM3ControlSim/Rigid Body1/Hydrodynamic Body/Wave Diffraction and Excitation Force Calculation/Linear Wave Excitation Force Variant Subsystem/Irregular Wave Excitation Force/MATLAB Function ==
  data: A input; Fext output; w input; fExtRE input; fExtIM input; phaseRand input; dw input; time input
function Fext = fcn(A,w,fExtRE,fExtIM,phaseRand,dw,time)
%#codegen

persistent A1 B1 B11 C1 D1 D11 E1 E11

A1=bsxfun(@plus,w*time,pi/2);
B1= sin(bsxfun(@plus,A1,phaseRand));
B11 = sin(bsxfun(@plus,w*time,phaseRand));
C1 = sqrt(bsxfun(@times,A,dw));
D1 =bsxfun(@times,fExtRE,C1);
D11 = bsxfun(@times,fExtIM,C1);
E1 = bsxfun(@times,B1,D1);
E11 = bsxfun(@times,B11,D11);

Fext = sum(bsxfun(@minus,E1,E11));

== matlab function RM3ControlSim/Rigid Body/Hydrodynamic Body/Structure/Motion Sensor/Angle ==
  data: Q input; E output
function E  = EulerAngle(Q)
% Euler Angle Type II or Tait-Bryan Angle for sequence 321 or zyx (Nautical or Cardan angles).
% Yaw [-180,180], followed by pitch [-90,90], followed by roll [-180,180]
E = zeros(3,1);
E(1) = atan2((2*(Q(1)*Q(2)+Q(3)*Q(4))),(1-2*(Q(2)^2+Q(3)^2)));
E(2) = asin(2*(Q(1)*Q(3)-Q(4)*Q(2)));
E(3) = atan2((2*(Q(1)*Q(4)+Q(2)*Q(3))),(1-2*(Q(3)^2+Q(4)^2)));

== matlab function RM3ControlSim/Rigid Body1/Hydrodynamic Body/Wave Diffraction and Excitation Force Calculation/Nonlinear FK Force Variant Subsystem/With Nonlinear FroudeKrylov Force/Diffraction and Excitation Forces ==
  data: x input; elv input; center input; f output; tnorm input; area input; rho input; g input; cg input; AH input; w input; dw input; wDepth input; deepWaterWave input; k input; typeNum input; t input; phaseRand input; wp output; wpMeanFS output; dt input; dtFe input
function [f, wp, wpMeanFS]  = nonFKForce(x,elv,center,tnorm,area,rho,g,cg,AH,w,dw,wDepth,deepWaterWave,k,typeNum,t,phaseRand, dt, dtFe)
    % Function to calculate wave exitation force and moment on a triangulated surface
    % NOTE: This function assumes that the STL file is imported with its CG at 0,0,0
    
    % Logic to calculate nonFKForce at reduced sample time
    persistent oldForce
    persistent oldWp
    persistent oldWpMeanFs
    
    if isempty(oldForce)
        [f, wp, wpMeanFS] = calc_force(x,elv,center,tnorm,area,rho,g,cg,AH,w,dw,wDepth,deepWaterWave,k,typeNum,t,phaseRand);
        oldForce = f;
        oldWp = wp;
        oldWpMeanFs = wpMeanFS;
    else
        if mod(t, dtFe) < dt/2
            [f, wp, wpMeanFS] = calc_force(x,elv,center,tnorm,area,rho,g,cg,AH,w,dw,wDepth,deepWaterWave,k,typeNum,t,phaseRand);
            oldForce = f;
            oldWp = wp;
            oldWpMeanFs = wpMeanFS;
        else
            f = oldForce;
            wp = oldWp;
            wpMeanFS = oldWpMeanFs;
        end
    end
end

function [f, wp, wpMeanFS]  = calc_force(x,elv,center,tnorm,area,rho,g,cg,AH,w,dw,wDepth,deepWaterWave,k,typeNum,t,phaseRand)
    % Function to apply translation and rotation, and calculate forces.
    
    % Compute new tri coords after cog rotation and translation
    centerMeanFS = offsetXYZ(center,cg);
    avMeanFS     = tnorm .* [area area area];
    
    % Compute new tri coords after cog rotation and translation
    center = rotateXYZ(center,[1 0 0],x(4));
    center = rotateXYZ(center,[0 1 0],x(5));
    center = rotateXYZ(center,[0 0 1],x(6));
    center = offsetXYZ(center,x);
    center = offsetXYZ(center,cg);
    % Compute new normal vectors coords after cog rotation and translation
    tnorm = rotateXYZ(tnorm,[1 0 0],x(4));
    tnorm = rotateXYZ(tnorm,[0 1 0],x(5));
    tnorm = rotateXYZ(tnorm,[0 0 1],x(6));
    
    % Copute area vectors
    av = tnorm .* [area area area];
    
    % Calculate the free surface
    wpMeanFS=pDis(centerMeanFS,       0,AH,w,dw,wDepth,deepWaterWave,t,k,phaseRand,typeNum,rho,g);
    wp      =pDis(center      ,     elv,AH,w,dw,wDepth,deepWaterWave,t,k,phaseRand,typeNum,rho,g);
    
    % Calculate forces
    f_linear   =FK(centerMeanFS,       cg,avMeanFS,wpMeanFS);
    f_nonLinear=FK(center      ,x(1:3)+cg,av      ,wp      ); 
    f = f_nonLinear-f_linear;
end

function verts = offsetXYZ(verts,x)
    % Function to move the position vertices
    verts(:,1) = verts(:,1) + x(1);
    verts(:,2) = verts(:,2) + x(2);
    verts(:,3) = verts(:,3) + x(3);
end

function xn = rotateXYZ(x,ax,t)
	% Function to rotate a point about an arbitrary axis
	% x: 3-componenet coordinates
	% ax: axis about which to rotate (must be a vector length 1)
	% t: rotation angle
	% xn: new coordinates after rotation
	rotMat = zeros(3);
	rotMat(1,1) = ax(1)*ax(1)*(1-cos(t))    + cos(t);
	rotMat(1,2) = ax(2)*ax(1)*(1-cos(t))    + ax(3)*sin(t);
	rotMat(1,3) = ax(3)*ax(1)*(1-cos(t))    - ax(2)*sin(t);
	rotMat(2,1) = ax(1)*ax(2)*(1-cos(t))    - ax(3)*sin(t);
	rotMat(2,2) = ax(2)*ax(2)*(1-cos(t))    + cos(t);
	rotMat(2,3) = ax(3)*ax(2)*(1-cos(t))    + ax(1)*sin(t);
	rotMat(3,1) = ax(1)*ax(3)*(1-cos(t))    + ax(2)*sin(t);
	rotMat(3,2) = ax(2)*ax(3)*(1-cos(t))    - ax(1)*sin(t);
	rotMat(3,3) = ax(3)*ax(3)*(1-cos(t))    + cos(t);
	xn = x*rotMat;
end

function f=pDis(center,elv,AH,w,dw,wDepth,deepWaterWave,t,k,phaseRand,typeNum,rho,g)
    % Function to calculate pressure distribution
    f = zeros(length(center(:,3)),1);
    z=zeros(length(center(:,1)),1);
    if typeNum <10
    elseif typeNum <20
        f = rho.*g.*AH(1).*cos(k(1).*center(:,1)-w(1)*t);
        if deepWaterWave == 0
            z=(center(:,3)-elv).*wDepth./(wDepth+elv);
            f = f.*(cosh(k(1).*(z+wDepth))./cosh(k(1)*wDepth));
        else
            z=(center(:,3)-elv);
            f = f.*exp(k(1).*z);
        end
    elseif typeNum <30
        for i=1:length(AH)
            if deepWaterWave == 0 && wDepth <= 0.5*pi/k(i)
                z=(center(:,3)-elv).*wDepth./(wDepth+elv);
                f_tmp = rho.*g.*sqrt(AH(i)*dw).*cos(k(i).*center(:,1)-w(i)*t-phaseRand(i));
                f = f + f_tmp.*(cosh(k(i).*(z+wDepth))./cosh(k(i).*wDepth));
            else
                z=(center(:,3)-elv);
                f_tmp = rho.*g.*sqrt(AH(i)*dw).*cos(k(i).*center(:,1)-w(i)*t-phaseRand(i));
                f = f + f_tmp.*exp(k(i).*z);
            end
        end
    end
    f(z>0)=0;
end

function f = FK(center,instcg,av,wp)
    % Function to calculate the force and moment about the cog due to Froude-Krylov pressure
    f = zeros(6,1);
    
    % Calculate the hydrostatic pressure at each triangle center
    pressureVect = [wp wp wp].*-av;
    
    % Compute force about cog
    f(1:3) = sum(pressureVect);
    
    % Compute moment about cog
    tmp1 = ones(length(center(:,1)),1);
    tmp2 = tmp1*instcg';
    center2cgVec = center-tmp2;
    
    f(4:6)= sum(cross(center2cgVec,pressureVect));
end

== matlab function RM3ControlSim/Rigid Body1/Hydrodynamic Body/Morrison Element and ViscousDampingForceCalculation/Morrison Element Variant Subsystem/Morrison Element On/Regular Wave Morison Force/MorrisonElements/OrbitalVelocity/MATLAB Function ==
  data: u output; v output; disp input size=[1 3]; waveNumber input size=[1 1]; waveFreq input size=[1 1]; waveAmp input size=[1 1]; randPhase input; time input; rampT input size=[1 1]; waveDir input size=[1 1]; waterDepth input size=[1 1]; g input size=[1 1]; w output; xa output; ya output; za output
function [u,v,w,xa,ya,za] = calc_orbital_vel(disp, waveNumber, waveFreq, waveAmp, randPhase, time, rampT, waveDir, waterDepth, g)
%#codegen

[u,v,w,xa,ya,za] = orbital_velocity(disp, waveNumber, waveFreq, waveAmp, randPhase, time, rampT, waveDir, waterDepth, g);

== matlab function RM3ControlSim/Rigid Body/Hydrodynamic Body/Wave Radiation Forces Calculation/SS CI and Constant-Damping-CoeVariant Subsystem/Convolution Integral Calculation/MATLAB Function ==
  data: v input double size=[6 1]; F_FM output double size=[6 1]; IRKB parameter double; lenJ parameter double size=1; CTTime parameter double
function F_FM = ConvolutionIntegral_interp(v, IRKB, lenJ, CTTime)
%#codegen
% Function to calculate convolution integral

%define persistent variables
interp_factor = 1;
persistent velocity IRKB_interp CTTime_interp;

if isempty(velocity) 
    CTTime_interp  = CTTime(1:interp_factor:end);
    velocity       = zeros(lenJ,length(CTTime_interp));
    IRKB_reordered = permute(IRKB,[3 1 2]);
    IRKB_interp    = IRKB_reordered(:,1:interp_factor:end, :);
end 
% shift velocity
velocity      = circshift(velocity, 1, 2);
velocity(:,1) = v(:);
%integrate

time_series = bsxfun(@times, IRKB_interp, velocity);
F_FM = squeeze(trapz(CTTime_interp,sum(time_series, 1)));

end
